simulink library "lib_subframe"  (R2021b)
settings: Solver=VariableStepAuto  StartTime=0.0  StopTime=10.0  RelTol=1e-3
libraries: slrealtimeutilitieslib x1
settings Model: Creator=jiw19031  LastModifiedBy=jiw19031

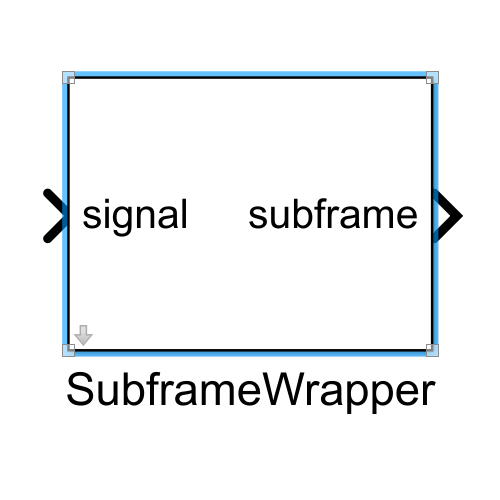
[thumbnail: Simulink's stored preview of the top-level diagram]
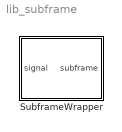
== system lib_subframe ==
  SubframeWrapper : Subsystem  mask{data_id=1}

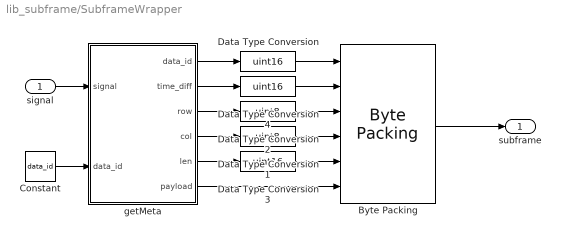
== system lib_subframe/SubframeWrapper ==
  signal : Inport
  "Byte Packing " : slrealtimeutilitieslib/Byte Packing  MaskPackedDataType=uint8  MaskUnpackedDataTypes={'uint16','uint16','uint8','uint8','uint16','double'}  MaskAlignment=1
  Constant : Constant  Value=data_id
  Data Type Conversion : DataTypeConversion  OutDataTypeStr=uint16
  Data Type Conversion1 : DataTypeConversion  OutDataTypeStr=uint8
  Data Type Conversion2 : DataTypeConversion  OutDataTypeStr=uint8
  Data Type Conversion3 : DataTypeConversion  OutDataTypeStr=uint16
  Data Type Conversion4 : DataTypeConversion  OutDataTypeStr=uint16
  getMeta : MATLAB Function  TreatAsAtomicUnit=on
  subframe : Outport
  wires:
  getMeta/1(data_id) -> Data Type Conversion/1
  signal/1 -> getMeta/1(signal)
  Data Type Conversion/1 -> "Byte Packing "/1
  getMeta/6(payload) -> "Byte Packing "/6
  "Byte Packing "/1 -> subframe/1
  Constant/1 -> getMeta/2("data_id ")
  getMeta/4(col) -> Data Type Conversion1/1
  Data Type Conversion1/1 -> "Byte Packing "/4
  getMeta/3(row) -> Data Type Conversion2/1
  Data Type Conversion2/1 -> "Byte Packing "/3
  getMeta/2(time_diff) -> Data Type Conversion4/1
  Data Type Conversion4/1 -> "Byte Packing "/2
  getMeta/5(len) -> Data Type Conversion3/1
  Data Type Conversion3/1 -> "Byte Packing "/5

== matlab function lib_subframe/SubframeWrapper/getMeta ==
  data: data_id output; time_diff output; row output; col output; len output; signal input; payload output; data_id input
function [ data_id,time_diff,row,col,len, payload]=get_meta(signal, data_id)
[row, col]=size(signal);
len = row*col;
time_diff = 0;
payload = signal;
